simulink model "State"  (R2019b)
settings: Solver=VariableStepAuto  StartTime=0.0  StopTime=10.0  RelTol=1e-3
settings Model: Creator=visha  LastModifiedBy=visha
settings OptimizationCC: DefaultParameterBehavior=Inlined

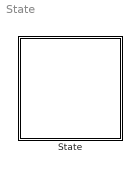
== system State ==
  State : Stateflow chart  BlockKeywords=__PRM__SERIALIZED__DATA__:Stateflow Chart,Stateflow Diagram  TreatAsAtomicUnit=on

== stateflow chart State/State ==
  state ON
  state OFF
  state RESET
  (default) -> ON
  RESET -> ON
  OFF -> ON [order 1]
  ON -> OFF
  OFF -> RESET [order 2]
